simulink library "Geartrain_Lib"  (Simulink 7.9)
settings: Solver=ode45  StartTime=0.0  StopTime=10.0  RelTol=1e-3
undefined symbols (not defined in the file): WT_Params
libraries: fl_lib x8, sdl_lib x3, nesl_utility x2, Geartrain_Lib x1, Brakes_Lib x1
Description:
  | Copyright 2011 MathWorks, Inc.
settings Model: Creator=smiller  LastModifiedBy=smiller

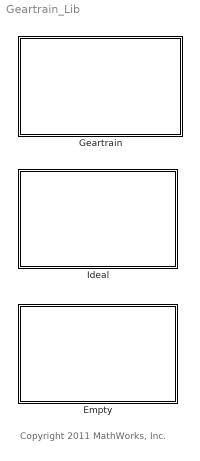
== system Geartrain_Lib ==
  note: Copyright 2011 MathWorks, Inc.
  Empty : Subsystem
      mask Display: image(imread('Geartrain_Empty_IMAGE.jpg'));
  Geartrain : Subsystem  BlockChoice=Empty
      settings: TemplateBlock=self  MemberBlocks=Empty,Ideal
  Ideal : Subsystem
      mask Display: image(imread('Geartrain_Ideal_IMAGE.jpg'));

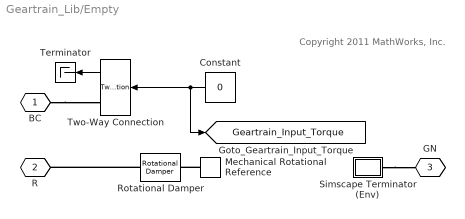
== system Geartrain_Lib/Empty ==
  note: Copyright 2011 MathWorks, Inc.
  Constant : Constant  Value=0
  Mechanical Rotational Reference : fl_lib/Mechanical/Rotational Elements/Mechanical Rotational Reference  SystemSampleTime=-1  t_Log=off  LocalVarNames=|t  LocalVarDescs=|t  LocalVarLogging=0
  Rotational Damper : fl_lib/Mechanical/Rotational Elements/Rotational Damper  D=WT_Params.Empty_Geartrain.damping N*m/(rad/s)  t_Log=off  w_Log=off  LocalVarNames=|t|w  LocalVarDescs=|t|w  LocalVarLogging=[0 0]
  Simscape Terminator (Env) : Subsystem
      mask Display:
      | plot([0 0.9],[0.5 0.5]);
      | plot([0.5 0.9],[0.3 0.3]);
      | plot([0.5 0.9],[0.7 0.7]);
      | plot([0.9 0.9],[0.7 0.3]);
  Terminator : Terminator
  Two-Way Connection : TwoWayConnection
  BC : PMIOPort  Tag=PMCPort  Port=1  Side=Left
  R : PMIOPort  Tag=PMCPort  Port=2  Side=Left
  GN : PMIOPort  Tag=PMCPort  Port=3  Side=Right
  tag scope: Geartrain_Input_Torque=global
  wires:
  Two-Way Connection/1 -> Terminator/1
  Constant/1 -> Two-Way Connection/1, [Geartrain_Input_Torque]
  connections:
  BC/RConn1 -- Two-Way Connection/RConn1
  Simscape Terminator (Env)/LConn1 -- GN/RConn1
  Rotational Damper/LConn1 -- R/RConn1
  Mechanical Rotational Reference/LConn1 -- Rotational Damper/RConn1

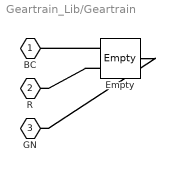
== system Geartrain_Lib/Geartrain ==
  Empty : Geartrain_Lib/Empty  SystemSampleTime=-1
  BC : PMIOPort  Port=1  Side=Left
  R : PMIOPort  Port=2  Side=Left
  GN : PMIOPort  Port=3  Side=Right
  connections:
  Empty/LConn1 -- BC/RConn1
  Empty/LConn2 -- R/RConn1
  Empty/RConn1 -- GN/RConn1

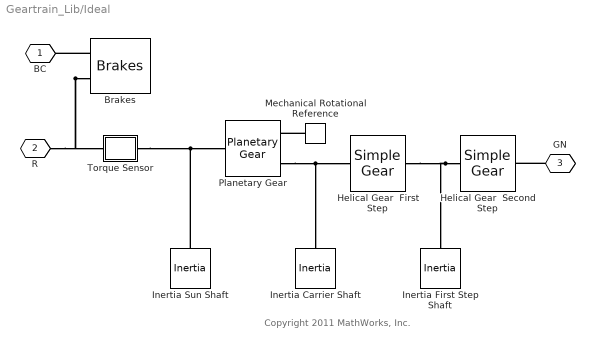
== system Geartrain_Lib/Ideal ==
  note: Copyright 2011 MathWorks, Inc.
  Brakes : Brakes_Lib/Brakes  SystemSampleTime=-1
  Helical Gear  First Step : sdl_lib/Gears/Simple Gear  SystemSampleTime=-1  ratio=WT_Params.Geartrain.Gear_Ratio.first_step  rotation_direction=2  friction_model=1  T_noload=0.1 N*m  T_nom=5 N*m  efficiency_nom=0.8  efficiency=0.8  mu_visc=[ 0 0 ] N*m/(rad/s)  w_thr=0.01 rad/s  LocalVarLogging=[]
  Helical Gear  Second Step : sdl_lib/Gears/Simple Gear  ratio=WT_Params.Geartrain.Gear_Ratio.second_step_primary_generator  rotation_direction=2  friction_model=1  T_noload=0.1 N*m  T_nom=5 N*m  efficiency_nom=0.8  efficiency=0.8  mu_visc=[ 0 0 ] N*m/(rad/s)  w_thr=0.01 rad/s  LocalVarLogging=[]
  Inertia Carrier Shaft : fl_lib/Mechanical/Rotational Elements/Inertia  SystemSampleTime=-1  inertia=WT_Params.Geartrain.inertia_sun_shaft kg*m^2  initial_velocity=0 rad/s  t_Log=off  LocalVarNames=|t  LocalVarDescs=|t  LocalVarLogging=0
  Inertia First Step Shaft : fl_lib/Mechanical/Rotational Elements/Inertia  SystemSampleTime=-1  inertia=WT_Params.Geartrain.inertia_first_step_shaft kg*m^2  initial_velocity=0 rad/s  t_Log=off  LocalVarNames=|t  LocalVarDescs=|t  LocalVarLogging=0
  Inertia Sun Shaft : fl_lib/Mechanical/Rotational Elements/Inertia  SystemSampleTime=-1  inertia=WT_Params.Geartrain.inertia_sun_shaft kg*m^2  initial_velocity=0 rad/s  t_Log=off  LocalVarNames=|t  LocalVarDescs=|t  LocalVarLogging=0
  Mechanical Rotational Reference : fl_lib/Mechanical/Rotational Elements/Mechanical Rotational Reference  SystemSampleTime=-1  t_Log=off  LocalVarNames=|t  LocalVarDescs=|t  LocalVarLogging=0
  Planetary Gear : sdl_lib/Gears/Planetary Gear  SystemSampleTime=-1  rs_ratio=WT_Params.Geartrain.Gear_Ratio.planetary  friction_model=1  efficiency=[ 0.96 0.98 ]  mu_visc=WT_Params.Geartrain.Planetary.viscous_losses N*m/(rad/s)  w_thr=[ 0.01 0.01 ] rad/s  LocalVarLogging=[]
  Torque Sensor : Subsystem
      mask Display: disp('S');
  BC : PMIOPort  Tag=PMCPort  Port=1  Side=Left
  R : PMIOPort  Tag=PMCPort  Port=2  Side=Left
  GN : PMIOPort  Tag=PMCPort  Port=3  Side=Right
  connections:
  Planetary Gear/RConn2 -- Helical Gear  First Step/RConn1 -- Inertia Carrier Shaft/LConn1
  Helical Gear  Second Step/RConn1 -- Helical Gear  First Step/LConn1 -- Inertia First Step Shaft/LConn1
  Inertia Sun Shaft/LConn1 -- Planetary Gear/LConn1 -- Torque Sensor/RConn1
  Mechanical Rotational Reference/LConn1 -- Planetary Gear/RConn1
  Brakes/LConn2 -- R/RConn1 -- Torque Sensor/LConn1
  Brakes/LConn1 -- BC/RConn1
  GN/RConn1 -- Helical Gear  Second Step/LConn1

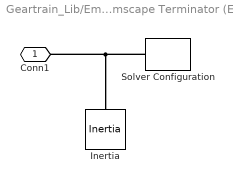
== system Geartrain_Lib/Empty/Simscape Terminator (Env) ==
  Inertia : fl_lib/Mechanical/Rotational Elements/Inertia  inertia=1.5e-3 kg*m^2  initial_velocity=0 rad/s  t_Log=off  LocalVarNames=|t  LocalVarDescs=|t  LocalVarLogging=0
  Solver Configuration : nesl_utility/Solver Configuration  PhysicalDomain=network_engine_domain  LeftPortType=input  RightPortType=generic  SubClassName=solver  UseCustomDae=off  DoDC=off  ResidualTolerance=1e-9  UseLocalSolver=off  LocalSolverChoice=NE_BACKWARD_EULER_ADVANCER  LocalSolverSampleTime=.001  DoFixedCost=off  MaxNonlinIter=3  MaxModeIter=2  LinearAlgebra=Sparse  Accelerate=off  Profile=off  UseLocalSampling=off  DelaysMemoryBudget=1024
  Conn1 : PMIOPort  Port=1  Side=Left
  connections:
  Solver Configuration/RConn1 -- Conn1/RConn1 -- Inertia/LConn1

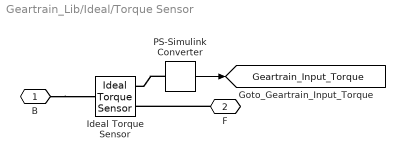
== system Geartrain_Lib/Ideal/Torque Sensor ==
  Ideal Torque Sensor : fl_lib/Mechanical/Mechanical Sensors/Ideal Torque Sensor  w_Log=off  t_Log=off  LocalVarNames=|w|t  LocalVarDescs=|w|t  LocalVarLogging=[0 0]
  PS-Simulink Converter : nesl_utility/PS-Simulink Converter  SystemSampleTime=-1  PhysicalDomain=network_engine_domain  LeftPortType=input  RightPortType=output  SubClassName=ps_output  Unit=1  AffineConversion=off
  B : PMIOPort  Port=1  Side=Left
  F : PMIOPort  Port=2  Side=Right
  tag scope: Geartrain_Input_Torque=global
  wires:
  PS-Simulink Converter/1 -> [Geartrain_Input_Torque]
  connections:
  B/RConn1 -- Ideal Torque Sensor/LConn1
  F/RConn1 -- Ideal Torque Sensor/RConn1
  PS-Simulink Converter/LConn1 -- Ideal Torque Sensor/RConn2
